simulink model "qubeLQGR_discrete_upwards"  (R2021b)
settings: Solver=ode1  StartTime=0.0  StopTime=120  RelTol=1e-3  EnableMultiTasking=on
values from neighbouring files (symbols this model uses):
  epsilon = 0.00242    [Controller_Dashboard.m]    (also in MPC_controller.m; MPC_controller_testing.m; max_structure_MPC_controller_testing.m)
  h = 0.01    [Controller_Dashboard.m]    (also in Design_of_nonlinear_controller.m = g4*D*alpha - g3*D*theta; MPC_controller.m; MPC_controller_testing.m; max_structure_MPC_controller_testing.m)
undefined symbols (not defined in the file or in its folder): Discrete, Humusoft, MF634, Time
libraries: sldrtlib x2, simulink x2, ctrlSharedLib x1
settings Model: Creator=rbabuska  LastModifiedBy=wpanijhuis
settings SolverCC: AlgebraicLoopSolver=TrustRegion
settings DataIOCC: LimitDataPoints=on  SaveFormat=Array  SignalLoggingSaveFormat=ModelDataLogs  ReturnWorkspaceOutputs=off
settings OptimizationCC: ExpressionDepthLimit=2147483647  LifeSpan=inf
settings DebuggingCC: UnderspecifiedInitializationDetection=Classic  MergeDetectMultiDrivingBlocksExec=none  FcnCallInpInsideContextMsg=warning  StateNameClashWarn=warning  SFUnexpectedBacktrackingDiag=warning  SFNoUnconditionalDefaultTransitionDiag=warning  SFExecutionAtInitializationDiag=none  SFMachineParentedDataDiag=warning  ArithmeticOperatorsInVariantConditions=warning
settings HardwareCC: ProdBitPerPointer=32  ProdBitPerSizeT=32  ProdBitPerPtrDiffT=32  ProdLargestAtomicFloat=None  ProdIntDivRoundTo=Undefined  ProdEndianess=Unspecified  ProdWordSize=32  ProdHWDeviceType=32-bit Generic
settings ModelReferenceCC: PropagateSignalLabelsOutOfModel=off
settings SFSimCC: SimUseLocalCustomCode=off  CustomCodeUndefinedFunction=UseInterfaceOnly
settings RTWCC: RTWUseLocalCustomCode=off
settings CodeAppCC: StateflowObjectComments=on
settings GRTTargetCC: TargetLangStandard=C89/C90 (ANSI)  CombineOutputUpdateFcns=off  GRTInterface=on
settings ConfigComp: CovMetricSettings=dw  CovSaveCumulativeToWorkspaceVar=on  CovSaveSingleToWorkspaceVar=on  CovExternalEMLEnable=off  CovSFcnEnable=off

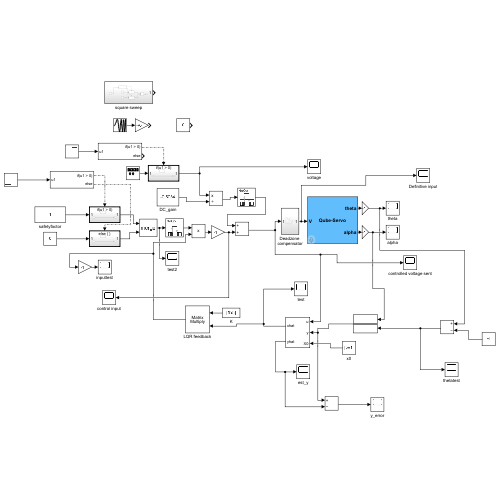
[thumbnail: Simulink's stored preview of the top-level diagram]
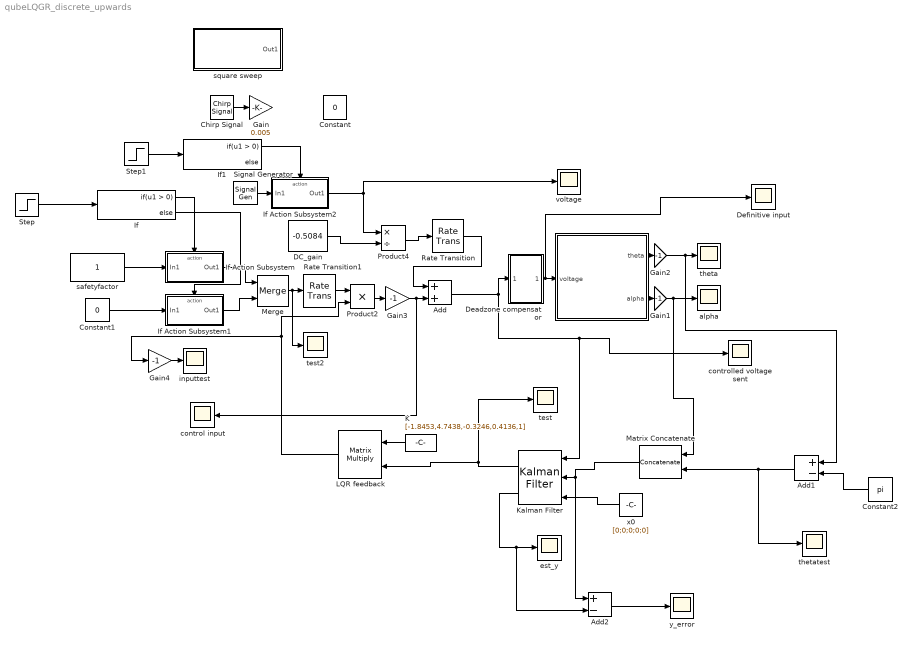
== system qubeLQGR_discrete_upwards ==
  " " : Subsystem  LoadFcn=hwinit  InitFcn=hwinit  mask{h=h}
      mask prompts: h "Sampling period [s]"
      mask Display:
      | disp('Qube-Servo')
      | port_label('output',1,'theta')
      | port_label('output',2,'alpha')
      | port_label('input',1,'V')
  Add : Sum  RndMeth=Nearest
  Add1 : Sum  Inputs=+-
  Add2 : Sum  Inputs=+-
  Chirp Signal : simulink/Sources/Chirp Signal  f1=1  T=120  f2=4
  Constant : Constant  Value=0
  Constant1 : Constant  Value=0
  Constant2 : Constant  Value=pi
  DC_gain : Constant  Value=-0.5084  SampleTime=h
  Deadzone compensator : Subsystem
  Definitive input : Scope
  Gain : Gain  Gain=0.005
  Gain{1..4} (4 alike) : Gain  Gain=-1
  If : If
  If Action Subsystem : Subsystem  TreatAsAtomicUnit=on
  If Action Subsystem1 : Subsystem  TreatAsAtomicUnit=on
  If Action Subsystem2 : Subsystem  TreatAsAtomicUnit=on
  If1 : If
  K : Constant  Value=[-1.8453,4.7438,-0.3246,0.4136,1]  VectorParams1D=off  SampleTime=h
  Kalman Filter : ctrlSharedLib/Kalman Filter  TimeDomain=Discrete-Time  UseCurrentEstimator=on  ModelSource=Individual A, B, C, D matrices  ModelSourceVariable=ss(0.95,1,1,0,1)  A=[0.9996,0.005906,0.00976,-0.00005518,0.1022;0.000003775,1.012,-0.0001249,0.009988,0.0961;-0.08811,1.168,0.9523,-0.008953,20.25;0.001128,2.431,-0.02479,1.002,19.14;0,0,0,0,1]  B=[0.1022;0.0961;20.25;19.14;0]  C=[1,0,0,0,0;0,1,0,0,0]  D=[0;0]  NumberOfStates=1  NumberOfInputs=1  NumberOfOutputs=1  InitialEstimateSource=Input port  X0=0  P0=10  UseK=off  UseGH=off  NumberOfProcessNoiseInputs=1  G=1  TimeInvariantG=on  H=0  TimeInvariantH=on  Q=blkdiag((1e-2)*eye(4), 1e-7)  TimeInvariantQ=on  R=1e-12  TimeInvariantR=on  N=0  TimeInvariantN=on  AddInputPort=on  AddEnablePort=off  OutputEstimatedY=on  OutputP=off  Ts=h
  LQR feedback : Product  Multiplication=Matrix(*)
  Matrix Concatenate : Concatenate  ConcatenateDimension=2
  Merge : Merge
  Product2 : Product
  Product4 : Product  Inputs=*/
  Rate Transition : RateTransition  OutPortSampleTime=h
  Rate Transition1 : RateTransition  OutPortSampleTime=h
  Signal Generator : SignalGenerator  WaveForm=square  Amplitude=0.05  Frequency=0.05
  Step : Step  Time=4  SampleTime=0
  Step1 : Step  Time=12  SampleTime=h
  alpha : Scope
  control input : Scope
  controlled voltage sent : Scope
  est_y : Scope
  inputtest : Scope
  safetyfactor : Constant  SampleTime=h
  square sweep : Subsystem
  test : Scope
  test2 : Scope
  theta : Scope
  thetatest : Scope
  voltage : Scope
  x0 : Constant  Value=[0;0;0;0;0]
  y_error : Scope
  wires:
  Matrix Concatenate/1 -> Add2/1, Kalman Filter/2
  K/1 -> LQR feedback/1
  Kalman Filter/1 -> test/1, LQR feedback/2
  If Action Subsystem/1(Out1) -> Merge/1
  Kalman Filter/2 -> Add2/2, est_y/1
  LQR feedback/1 -> Product2/2, Gain4/1
  DC_gain/1 -> Product4/2
  Product4/1 -> Rate Transition/1
  Deadzone compensator/1(Out1) -> Definitive input/1, " "/1(voltage)
  Gain1/1 -> Matrix Concatenate/1, alpha/1
  Gain2/1 -> Add1/1, theta/1
  If Action Subsystem2/1(Out1) -> voltage/1, Product4/1
  " "/2(alpha) -> Gain1/1
  " "/1(theta) -> Gain2/1
  Chirp Signal/1 -> Gain/1
  x0/1 -> Kalman Filter/3
  Product2/1 -> Gain3/1
  Gain3/1 -> control input/1, Add/2
  Rate Transition/1 -> Add/1
  Add/1 -> Deadzone compensator/1(In1), controlled voltage sent/1, Kalman Filter/1
  Step/1 -> If/1
  If/1 -> If Action Subsystem/Action
  safetyfactor/1 -> If Action Subsystem/1(In1)
  If/2 -> If Action Subsystem1/Action
  Constant1/1 -> If Action Subsystem1/1(In1)
  If Action Subsystem1/1(Out1) -> Merge/2
  Merge/1 -> test2/1, Rate Transition1/1
  Rate Transition1/1 -> Product2/1
  Add1/1 -> thetatest/1, Matrix Concatenate/2
  Constant2/1 -> Add1/2
  Add2/1 -> y_error/1
  Gain4/1 -> inputtest/1
  Step1/1 -> If1/1
  Signal Generator/1 -> If Action Subsystem2/1(In1)
  If1/1 -> If Action Subsystem2/Action

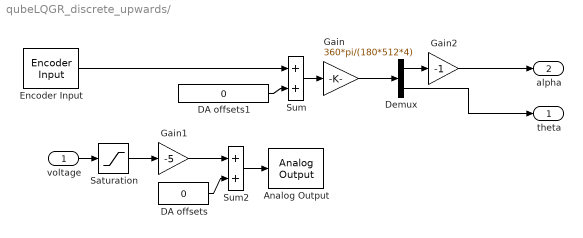
== system qubeLQGR_discrete_upwards/  ==
  voltage : Inport
  Analog Output : sldrtlib/Analog Output  SampleTime=h  MaxMissedTicks=100  ShowMissedTicks=off  YieldWhenWaiting=off  DrvName=Humusoft/MF634  DrvAddress=4294967295  DrvOptions=0  Channels=[1]  RangeMode=2  VoltRange=1  InitialValue=0  FinalValue=0
      settings: AttributesFormatString=Humusoft\nMF634 [auto]
  DA offsets : Constant  Value=0
  DA offsets1 : Constant  Value=0  SampleTime=h
  Demux : Demux  Outputs=2
  Encoder Input : sldrtlib/Encoder Input  SampleTime=h  MaxMissedTicks=100  ShowMissedTicks=off  YieldWhenWaiting=off  DrvName=Humusoft/MF634  DrvAddress=4294967295  DrvOptions=0  Channels=[1,2]  QuadMode=3  IndexPulse=1  InputFilter=Inf  DataType=1
      settings: AttributesFormatString=Humusoft\nMF634 [auto]
  Gain : Gain  Gain=360*pi/(180*512*4)  SaturateOnIntegerOverflow=on  OutDataTypeStr=Inherit: Same as input  ParamDataTypeStr=Inherit: Same as input
  Gain1 : Gain  Gain=-5  SaturateOnIntegerOverflow=on  OutDataTypeStr=Inherit: Same as input  ParamDataTypeStr=Inherit: Same as input
  Gain2 : Gain  Gain=-1  SaturateOnIntegerOverflow=on  OutDataTypeStr=Inherit: Same as input  ParamDataTypeStr=Inherit: Same as input
  Saturation : Saturate  UpperLimit=1  LowerLimit=-1
  Sum : Sum  InputSameDT=on  SaturateOnIntegerOverflow=on  OutDataTypeStr=Inherit: Same as first input
  Sum2 : Sum  InputSameDT=on  SaturateOnIntegerOverflow=on  OutDataTypeStr=Inherit: Same as first input
  theta : Outport  Tag=Cable length
  alpha : Outport  Tag=Cable length  Port=2
  wires:
  Sum/1 -> Gain/1
  DA offsets1/1 -> Sum/2
  Gain1/1 -> Sum2/1
  Sum2/1 -> Analog Output/1
  DA offsets/1 -> Sum2/2
  voltage/1 -> Saturation/1
  Encoder Input/1 -> Sum/1
  Saturation/1 -> Gain1/1
  Demux/1 -> Gain2/1
  Gain/1 -> Demux/1
  Gain2/1 -> alpha/1
  Demux/2 -> theta/1

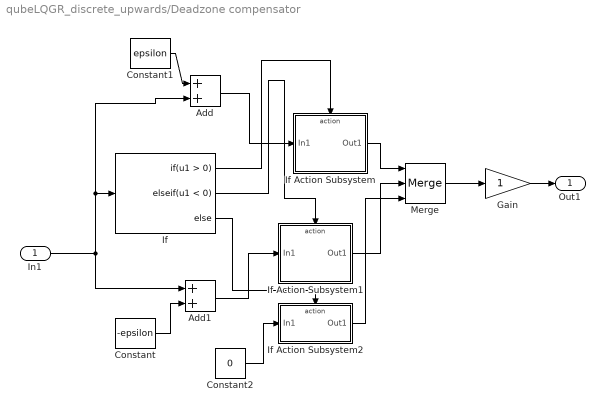
== system qubeLQGR_discrete_upwards/Deadzone compensator ==
  In1 : Inport
  Add : Sum
  Add1 : Sum
  Constant : Constant  Value=-epsilon
  Constant1 : Constant  Value=epsilon
  Constant2 : Constant  Value=0
  Gain : Gain
  If : If  ElseIfExpressions=u1 < 0
  If Action Subsystem : Subsystem  TreatAsAtomicUnit=on
  If Action Subsystem1 : Subsystem  TreatAsAtomicUnit=on
  If Action Subsystem2 : Subsystem  TreatAsAtomicUnit=on
  Merge : Merge  Inputs=3
  Out1 : Outport
  wires:
  If Action Subsystem/1(Out1) -> Merge/1
  Gain/1 -> Out1/1
  Merge/1 -> Gain/1
  If/2 -> If Action Subsystem1/Action
  Add/1 -> If Action Subsystem/1(In1)
  If/1 -> If Action Subsystem/Action
  If Action Subsystem1/1(Out1) -> Merge/2
  In1/1 -> Add1/1, Add/2, If/1
  Constant1/1 -> Add/1
  Constant/1 -> Add1/2
  Add1/1 -> If Action Subsystem1/1(In1)
  Constant2/1 -> If Action Subsystem2/1(In1)
  If/3 -> If Action Subsystem2/Action
  If Action Subsystem2/1(Out1) -> Merge/3

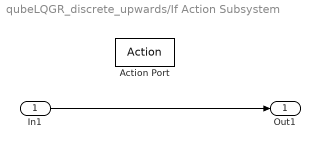
== system qubeLQGR_discrete_upwards/If Action Subsystem ==
  In1 : Inport
  Action Port : ActionPort  ActionPortLabel=if(u1 > 0)
  Out1 : Outport
  wires:
  In1/1 -> Out1/1

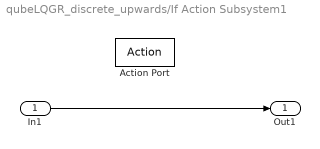
== system qubeLQGR_discrete_upwards/If Action Subsystem1 ==
  In1 : Inport
  Action Port : ActionPort  ActionPortLabel=else
  Out1 : Outport
  wires:
  In1/1 -> Out1/1

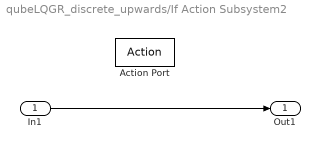
== system qubeLQGR_discrete_upwards/If Action Subsystem2 ==
  In1 : Inport
  Action Port : ActionPort  ActionPortLabel=if(u1 > 0)
  Out1 : Outport
  wires:
  In1/1 -> Out1/1

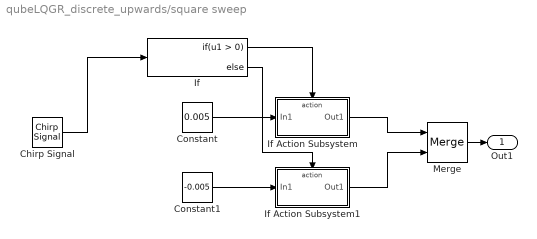
== system qubeLQGR_discrete_upwards/square sweep ==
  Chirp Signal : simulink/Sources/Chirp Signal  f1=0  T=120  f2=5
  Constant : Constant  Value=0.005
  Constant1 : Constant  Value=-0.005
  If : If
  If Action Subsystem : Subsystem  TreatAsAtomicUnit=on
  If Action Subsystem1 : Subsystem  TreatAsAtomicUnit=on
  Merge : Merge
  Out1 : Outport
  wires:
  Merge/1 -> Out1/1
  If/2 -> If Action Subsystem1/Action
  Chirp Signal/1 -> If/1
  Constant/1 -> If Action Subsystem/1(In1)
  If Action Subsystem1/1(Out1) -> Merge/2
  If Action Subsystem/1(Out1) -> Merge/1
  If/1 -> If Action Subsystem/Action
  Constant1/1 -> If Action Subsystem1/1(In1)

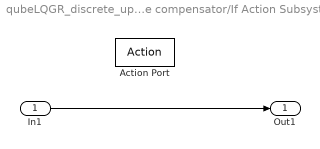
== system qubeLQGR_discrete_upwards/Deadzone compensator/If Action Subsystem ==
  In1 : Inport
  Action Port : ActionPort  ActionPortLabel=if(u1 > 0)
  Out1 : Outport
  wires:
  In1/1 -> Out1/1

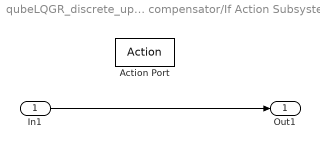
== system qubeLQGR_discrete_upwards/Deadzone compensator/If Action Subsystem1 ==
  In1 : Inport
  Action Port : ActionPort  ActionPortLabel=elseif(u1 < 0)
  Out1 : Outport
  wires:
  In1/1 -> Out1/1

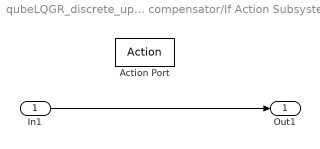
== system qubeLQGR_discrete_upwards/Deadzone compensator/If Action Subsystem2 ==
  In1 : Inport
  Action Port : ActionPort  ActionPortLabel=else
  Out1 : Outport
  wires:
  In1/1 -> Out1/1

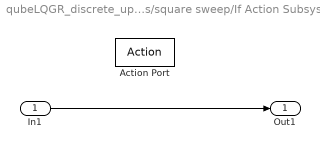
== system qubeLQGR_discrete_upwards/square sweep/If Action Subsystem ==
  In1 : Inport
  Action Port : ActionPort  ActionPortLabel=if(u1 > 0)
  Out1 : Outport
  wires:
  In1/1 -> Out1/1

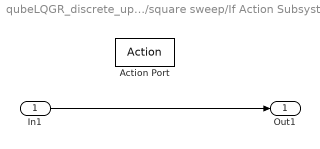
== system qubeLQGR_discrete_upwards/square sweep/If Action Subsystem1 ==
  In1 : Inport
  Action Port : ActionPort  ActionPortLabel=else
  Out1 : Outport
  wires:
  In1/1 -> Out1/1
